simulink model "TV"  (R2022b)
settings: Solver=ode1  StartTime=0.0  StopTime=30  FixedStep=Ts  RelTol=1e-3
PreLoadFcn:
  | run("Fzg_Par.m");
InitFcn:
  | run("Fzg_Par.m");
values from neighbouring files (symbols this model uses):
  c_alpha_H = 13400    [Fzg_Par.m]    (also in Fzg_par.m)
  c_alpha_V = 9300    [Fzg_Par.m]    (also in Fzg_par.m)
  delta_V = 36 * SAS    (= 29.52)    [Fzg_Par.m]    (also in Fzg_par.m = -1.01419878296)
  K_PD = 5    [Fzg_Par.m]
  L038_GPS_Speed = [44.3579978943 44.6180000305 44.8540000916 45.0340003967 45.2140007019 45.3940010071 45.5740013123 45.7659988403 45.986000061 46.2060012817 46.4259986877 46.6459999084 ... (1603 elements, 1603x1)]    [Lap38Data.mat]    (also in Testrunde_PATZE.mat = [33.5580024719 33.5380020142 33.5180015564 33.5099983215 33.)
  L038_LateralAcc = [-0.446329861879 -0.243792653084 -0.104723833501 -0.0600545369089 -0.108962662518 -0.216311529279 -0.338253945112 -0.428329110146 -0.43160328269 -0.432035714388 -0.438702851534 -0.456409007311 ... (1603 elements, 1603x1)]    [Lap38Data.mat]
  L038_SAS = [2.17868804932 8.86017131805 12.9289064407 10.9012298584 8.87355232239 6.84587574005 4.81819868088 2.60318017006 -0.0489690937102 -2.70111823082 -5.35326766968 -8.00541687012 ... (1603 elements, 1603x1)]    [Lap38Data.mat]    (also in Testrunde_PATZE.mat = [78.6100845337 74.5163192749 70.4225540161 66.6965942383 66.)
  L038_time = [0 0.019999999553 0.0399999991059 0.0599999986589 0.0799999982119 0.10000000149 0.119999997318 0.140000000596 0.159999996424 0.180000007153 0.20000000298 0.219999998808 ... (1603 elements, 1603x1)]    [Lap38Data.mat]    (also in Testrunde_PATZE.mat = [0 0.019999999553 0.0399999991059 0.0599999986589 0.07999999)
  L038_YawRate = [-40.4006690979 -35.1522026062 -28.5971374512 -21.3668518066 -14.4125385284 -8.49562072754 -3.29422926903 1.16192114353 2.16577601433 2.1207613945 0.961856245995 -1.21237790585 ... (1603 elements, 1603x1)]    [Lap38Data.mat]    (also in Testrunde_PATZE.mat = [70.8436279297 71.1428375244 71.3223114014 71.4394073486 71.)
  l_fzg = 1530/1000    (= 1.53)    [Fzg_Par.m]    (also in Fzg_par.m = 1.3)
  l_H_fzg = 507/1000    (= 0.507)    [Fzg_Par.m]    (also in Fzg_par.m)
  l_V_fzg = 1023/1000    (= 1.023)    [Fzg_Par.m]    (also in Fzg_par.m)
  m_fzg = 241.5 + 82    (= 323.5)    [Fzg_Par.m]    (also in Fzg_par.m)
  ss_A = [-(c_alpha_V*l_V_fzg^2+c_alpha_H*l_H_fzg^2)/(J_fzg_z*v_x) (c_alpha_H*l_H_fzg-c_alpha_V*l_V_fzg)/J_fzg_z ... (first row only)    [Fzg_Par.m]    (also in Fzg_par.m)
  ss_B = [(c_alpha_V*l_V_fzg)/J_fzg_z -(c_alpha_H*l_H_fzg)/J_fzg_z ... (first row only)    [Fzg_Par.m]    (also in Fzg_par.m)
  ss_C = [1 0]    [Fzg_Par.m]    (also in Fzg_par.m)
  ss_D = [0 0]    [Fzg_Par.m]    (also in Fzg_par.m)
  t_H_fzg = 1200/1000    (= 1.2)    [Fzg_par.m]
  T_p = T_v/10    (= 0.01)    [Fzg_Par.m]
  T_v = 0.1    [Fzg_Par.m]
  v_x = 30/3.6    (= 8.33333333333)    [Fzg_Par.m]    (also in Fzg_par.m = 10)
settings Model: Creator=shoot  LastModifiedBy=shoot

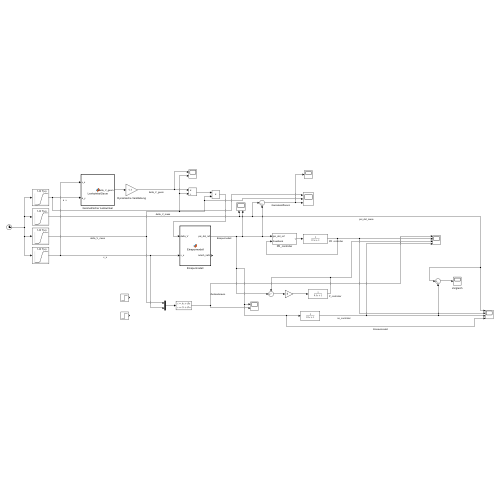
[thumbnail: Simulink's stored preview of the top-level diagram]
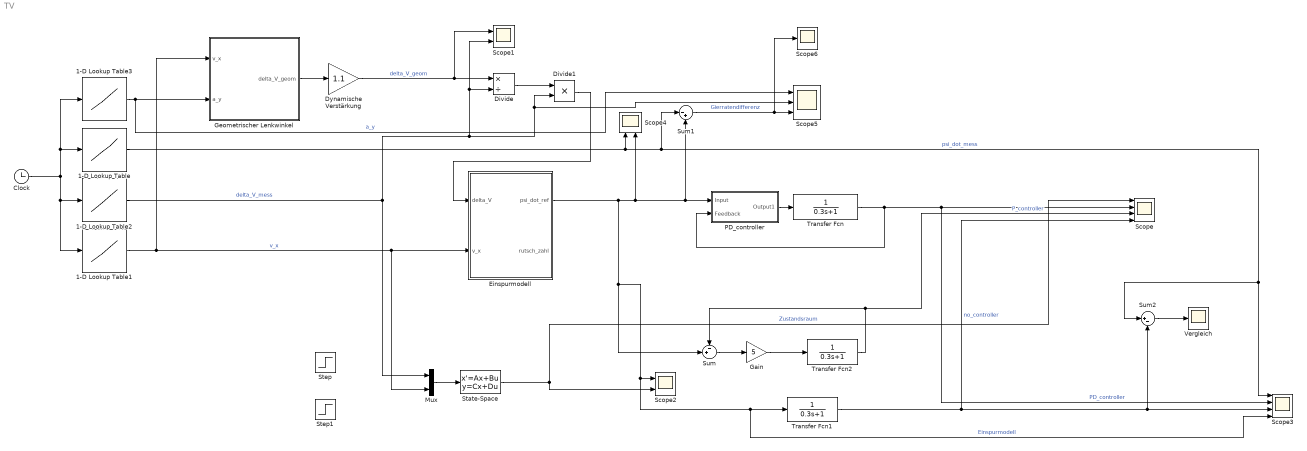
== system TV ==
  1-D Lookup Table : Lookup_n-D  NumberOfTableDimensions=1  BreakpointsForDimension1=L038_time  Table=L038_YawRate  InternalRulePriority=Speed  RndMeth=Simplest
  1-D Lookup Table1 : Lookup_n-D  NumberOfTableDimensions=1  BreakpointsForDimension1=L038_time  Table=L038_GPS_Speed/3.6  InternalRulePriority=Speed  RndMeth=Simplest
  1-D Lookup Table2 : Lookup_n-D  NumberOfTableDimensions=1  BreakpointsForDimension1=L038_time  Table=L038_SAS*0.29  InternalRulePriority=Speed  RndMeth=Simplest
  1-D Lookup Table3 : Lookup_n-D  NumberOfTableDimensions=1  BreakpointsForDimension1=L038_time  Table=L038_LateralAcc*9.81  InternalRulePriority=Speed  RndMeth=Simplest
  Clock : Clock
  Divide : Product  Inputs=*/
  Divide1 : Product  Inputs=**
  Dynamische Verstärkung : Gain  Gain=1.1
  Einspurmodell : MATLAB Function  TreatAsAtomicUnit=on
  Gain : Gain  Gain=5
  Geometrischer Lenkwinkel : MATLAB Function  TreatAsAtomicUnit=on
  Mux : Mux  Inputs=2
  PD_controller : Subsystem
  Scope : Scope  NumInputPorts=4
  Scope1 : Scope  NumInputPorts=2
  Scope2 : Scope  NumInputPorts=2
  Scope3 : Scope  NumInputPorts=4
  Scope4 : Scope  NumInputPorts=2
  Scope5 : Scope  NumInputPorts=3
  Scope6 : Scope
  State-Space : StateSpace  A=ss_A  B=ss_B  C=ss_C  D=ss_D  InitialCondition=0
  Step : Step  After=delta_V  SampleTime=0
  Step1 : Step  After=v_x  SampleTime=0
  Sum : Sum  Inputs=-+|
  Sum1 : Sum  Inputs=|-+
  Sum2 : Sum  Inputs=|+-
  Transfer Fcn : TransferFcn  Denominator=[0.3 1]
  Transfer Fcn1 : TransferFcn  Denominator=[0.3 1]
  Transfer Fcn2 : TransferFcn  Denominator=[0.3 1]
  Vergleich : Scope
  wires:
  Transfer Fcn1/1 -> Sum2/2, Scope3/3, Scope/4  "no_controller"
  PD_controller/1(Output1) -> Transfer Fcn/1
  Sum/1 -> Gain/1
  Gain/1 -> Transfer Fcn2/1
  Transfer Fcn2/1 -> Sum/1, Scope/3  "P_controller"
  Transfer Fcn/1 -> PD_controller/2(Feedback), Scope3/2, Scope/2  "PD_controller"
  Mux/1 -> State-Space/1
  State-Space/1 -> Scope/1, Scope2/2  "Zustandsraum"
  Clock/1 -> 1-D Lookup Table/1, 1-D Lookup Table3/1, 1-D Lookup Table2/1, 1-D Lookup Table1/1
  1-D Lookup Table/1 -> Sum1/1, Sum2/1, Scope3/1, Scope4/1  "psi_dot_mess"
  1-D Lookup Table1/1 -> Geometrischer Lenkwinkel/1(v_x), Mux/2, Einspurmodell/2(v_x)  "v_x"
  1-D Lookup Table2/1 -> Scope1/2, Divide/2, Divide1/2, Scope5/2, Mux/1  "delta_V_mess"
  Einspurmodell/1(psi_dot_ref) -> Scope2/1, Scope3/4, Transfer Fcn1/1, Sum/2, Sum1/2, PD_controller/1(Input), Scope4/2  "Einspurmodell"
  Sum2/1 -> Vergleich/1
  Geometrischer Lenkwinkel/1(delta_V_geom) -> Dynamische Verstärkung/1
  1-D Lookup Table3/1 -> Geometrischer Lenkwinkel/2(a_y), Scope5/1  "a_y"
  Dynamische Verstärkung/1 -> Scope1/1, Divide/1  "delta_V_geom"
  Divide/1 -> Divide1/1
  Divide1/1 -> Einspurmodell/1(delta_V)
  Sum1/1 -> Scope6/1, Scope5/3  "Gierratendifferenz"

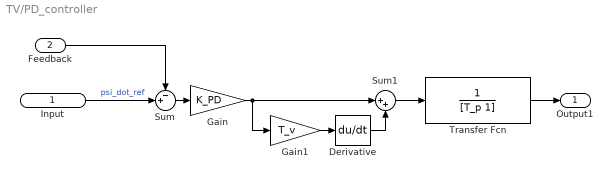
== system TV/PD_controller ==
  Input : Inport
  Feedback : Inport  Port=2
  Derivative : Derivative
  Gain : Gain  Gain=K_PD
  Gain1 : Gain  Gain=T_v
  Sum : Sum  Inputs=-+|
  Sum1 : Sum  Inputs=|++
  Transfer Fcn : TransferFcn  Denominator=[T_p 1]
  Output1 : Outport
  wires:
  Feedback/1 -> Sum/1
  Gain1/1 -> Derivative/1
  Sum1/1 -> Transfer Fcn/1
  Gain/1 -> Gain1/1, Sum1/1
  Input/1 -> Sum/2  "psi_dot_ref"
  Sum/1 -> Gain/1
  Derivative/1 -> Sum1/2
  Transfer Fcn/1 -> Output1/1

== matlab function TV/Geometrischer Lenkwinkel ==
  data: delta_V_geom output; v_x input; a_y input; t_H_fzg parameter; l_fzg parameter
function delta_V_geom  = LenkwinkelGeom(v_x,a_y, t_H_fzg, l_fzg)

    delta_V_geom = atand(l_fzg/((v_x*v_x/a_y)+(t_H_fzg/2)));

== matlab function TV/Einspurmodell ==
  data: psi_dot_ref output; delta_V input; v_x input; rutsch_zahl output; m_fzg parameter; l_fzg parameter; l_V_fzg parameter; l_H_fzg parameter; c_alpha_V parameter; c_alpha_H parameter
function [psi_dot_ref, rutsch_zahl]   = Einspurmodell(delta_V, v_x, m_fzg, l_fzg, l_V_fzg, l_H_fzg, c_alpha_V, c_alpha_H)
%#codegen

% Charakteristische Geschwindigkeit zum Quadrat
square_v_ch = c_alpha_V * c_alpha_H * l_fzg / (m_fzg * ((c_alpha_H * l_H_fzg) - (c_alpha_V * l_V_fzg)));

% Soll Gierrate
%psi_dot_ref = v_x * delta_V / (l_fzg * (1 + (v_x^2 / square_v_ch)));
psi_dot_ref = v_x * delta_V / l_fzg;

rutsch_zahl = v_x^2/square_v_ch;
end
